simulink model "Cont"  (R2021a)
settings: Solver=VariableStepAuto  StartTime=0.0  StopTime=10.0  RelTol=1e-3
settings Model: Creator=kmckell  LastModifiedBy=MikeyG

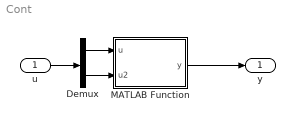
== system Cont ==
  u : Inport
  Demux : Demux  Outputs=2
  MATLAB Function : MATLAB Function  TreatAsAtomicUnit=on
  y : Outport
  wires:
  MATLAB Function/1(y) -> y/1
  u/1 -> Demux/1
  Demux/1 -> MATLAB Function/1(u)
  Demux/2 -> MATLAB Function/2(u2)

== matlab function Cont/MATLAB Function ==
  data: u input; y output; u2 input
function y = fcn(u, u2)

Ka     = 5.1793;     % Power Amplifier
N      = 8.1;        % Speed Reduction Factor
Kp     = 4.90379;    % Position Feedback Gain [V/rad]
Kt     = .1429;      % Tachometer Gain [V/rad/s]
u = u/Kp;
u2 = u2/Kt/N;

k = plus(plus(times(times(2,u),4.5),plus(u,u2)),plus(plus(plus(u2,plus(u,plus(plus(u,u2),times(-1,u2)))),times(-1,u2)),u));
y = -k/Ka;
